simulink library "lib_converters"  (R2020b)
settings: Solver=VariableStepAuto  StartTime=0.0  StopTime=10.0  RelTol=1e-3
undefined symbols (not defined in the file): C_sc, DiscIntNeverNeededParam
libraries: powerlib x170, simulink x12, $bdroot x6, powerlib_meascontrol x3
(part 1 of 3)
settings Model: Creator=maloc  LastModifiedBy=maloc

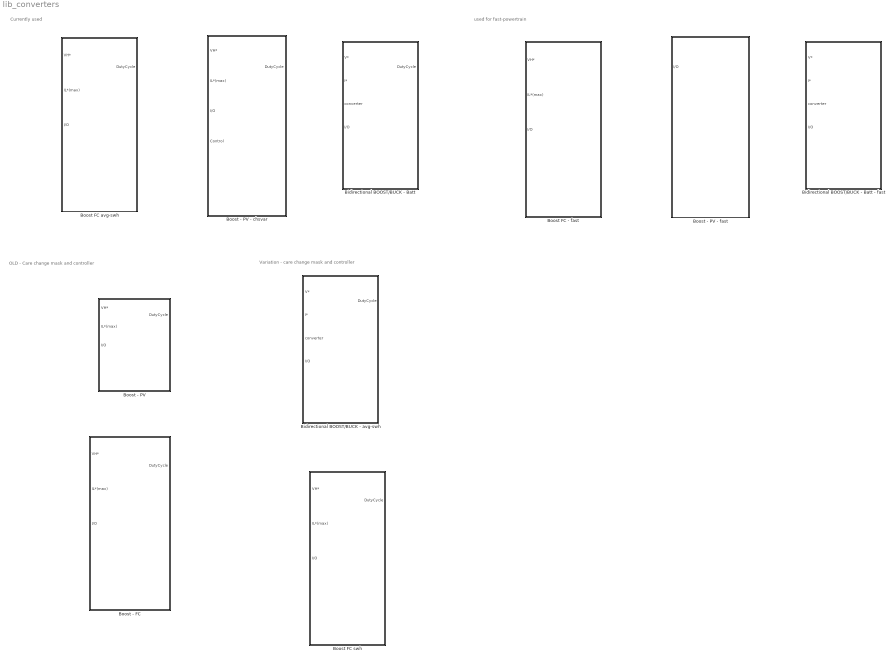
== system lib_converters ==
  note: Variation - care change mask and controller
  note: OLD - Care change mask and controller
  note: Currently used
  note: used for fast-powertrain
  Bidirectional BOOST/BUCK - Batt : Subsystem  mask(Average value DC/DC Bidirectional converter for Batt){n_buck=0.9, Tr_buck=1e-3, damp_buck=0, n_boost=0.9, Tr_boost=1e-3, damp_boost=0, max_curr=[45 -5], Co=1e-4, CL=1, Li=2e-3, Ts=1e-4}
      mask prompts: n_buck "Buck Efficiency [0,1]"; Tr_buck "Buck Regulator Response Time (s)"; damp_buck "Buck Damping ratio"; n_boost "Boost Efficiency [0,1]"; Tr_boost "Boost Regulator Response Time (s)"; damp_boost "Boost Damping ratio"; max_curr "Max currents [+ -] (A)"; Co "Capacitor (F)"; CL "DC Bus Capacitor (F)"; Li "Inductor (H)"; Ts "Sample Time (s)"
      mask help:
      | This block implements an average-value DC/DC Bidirectional boost/buck converter.
      | -> Boost
      | - V* is the voltage control variable. It controls the dc bus voltage (higher voltage part)
      | - I* is the current control variable. It controls the battery current (lower voltage part)
      |
      | <- Buck
      | - V* is the voltage control variable. It controls the battery voltage (lower voltage part)
      | - I* is the current control variable. It controls the current that comes from the dc bus (higher voltage part)
      |
      | - converter input controls the converter mode : 0 = Boost, 1 = Buck
      mask init:
      | L=Li; 
      | C=Co+CL;
      | 
      | 
      | 
      | %Buck :
      | %Current regulator
      | zetai_buck =damp_buck;
      | thau_si_buck =Tr_buck/10;
      | zetawni_buck=(-log(0.05*sqrt(1-zetai_buck^2)))/thau_si_buck;
      | Kpi_buck=2*L*zetawni_buck;
      | wni_buck=zetawni_buck/zetai_buck;
      | Kii_buck=L*wni_buck^2;
      |  
      | %Voltage regulator
      | zetav_buck=damp_buck;
      | thau_sv_buck=Tr_buck; %response time
      | zetawnv_buck=(-log(0.05*sqrt(1-zetav_buck^2)))/thau_sv_buck;
      | Kpv_buck=2*C*zetawnv_buck;
      | wnv_buck=zetawnv_buck/zetav_buck;
      | Kiv_buck=C*wnv_buck^2;
      | 
      | 
      | 
      | 
      | 
      | %Boost :
      | %Current regulator
      | zetai_boost=damp_boost;
      | thau_si_boost =Tr_boost/10; 
      | zetawni_boost =(-log(0.05*sqrt(1-zetai_boost ^2)))/thau_si_boost;
      | Kpi_boost=2*L*zetawni_boost;
      | wni_boost =zetawni_boost /zetai_boost;
      | Kii_boost=L*wni_boost ^2;
      |  
      | %Voltage regulator
      | zetav_boost =damp_boost;
      | thau_sv_boost =Tr_boost; %response time
      | zetawnv_boost =(-log(0.05*sqrt(1-zetav_boost ^2)))/thau_sv_boost;
      | Kpv_boost=2*C*zetawnv_boost;
      | wnv_boost =zetawnv_boost /zetav_boost;
      | Kiv_boost=C*wnv_boost ^2;
      mask Help:
      | 0 - Boost -->
      | <-- 1 - Buck
      mask DialogControl Container4 Prompt: Buck
      mask DialogControl Container5 Prompt: Boost
      mask DialogControl Container6 Prompt: All
  Bidirectional BOOST/BUCK - Batt - fast : Subsystem  AncestorBlock=lib_converters/Bidirectional BOOST//BUCK - Batt  mask(Average value DC/DC Bidirectional converter for Batt){n_buck=0.9, Tr_buck=1e-3, damp_buck=0, n_boost=0.9, Tr_boost=1e-3, damp_boost=0, max_curr=[45 -5], Co=1e-4, CL=1, Li=2e-3, Ts=1e-4}
      mask prompts: n_buck "Buck Efficiency [0,1]"; Tr_buck "Buck Regulator Response Time (s)"; damp_buck "Buck Damping ratio"; n_boost "Boost Efficiency [0,1]"; Tr_boost "Boost Regulator Response Time (s)"; damp_boost "Boost Damping ratio"; max_curr "Max currents [+ -] (A)"; Co "Capacitor (F)"; CL "DC Bus Capacitor (F)"; Li "Inductor (H)"; Ts "Sample Time (s)"
      mask help:
      | This block implements an average-value DC/DC Bidirectional boost/buck converter.
      | -> Boost
      | - V* is the voltage control variable. It controls the dc bus voltage (higher voltage part)
      | - I* is the current control variable. It controls the battery current (lower voltage part)
      |
      | <- Buck
      | - V* is the voltage control variable. It controls the battery voltage (lower voltage part)
      | - I* is the current control variable. It controls the current that comes from the dc bus (higher voltage part)
      |
      | - converter input controls the converter mode : 0 = Boost, 1 = Buck
      mask init: same as lib_converters/Bidirectional BOOST/BUCK - Batt
      mask Help:
      | 0 - Boost -->
      | <-- 1 - Buck
      mask DialogControl Container4 Prompt: Buck
      mask DialogControl Container5 Prompt: Boost
      mask DialogControl Container6 Prompt: All
  Bidirectional BOOST/BUCK - avg-swh : Subsystem  mask(Average value DC/DC Bidirectional converter for Batt){n_buck=0.9, Tr_buck=1e-3, n_boost=0.9, Tr_boost=1e-3, Co=1e-4, CL=1, Li=2e-3, Ts=1e-4}
      mask prompts: n_buck "Buck Efficiency [0,1]"; Tr_buck "Buck Regulator Response Time (s)"; n_boost "Boost Efficiency [0,1]"; Tr_boost "Boost Regulator Response Time (s)"; Co "Capacitor (F)"; CL "DC Bus Capacitor (F)"; Li "Inductor (H)"; Ts "Sample Time (s)"
      mask help:
      | This block implements an average-value DC/DC Bidirectional boost/buck converter.
      | -> Boost
      | - V* is the voltage control variable. It controls the dc bus voltage (higher voltage part)
      | - I* is the current control variable. It controls the battery current (lower voltage part)
      |
      | <- Buck
      | - V* is the voltage control variable. It controls the battery voltage (lower voltage part)
      | - I* is the current control variable. It controls the current that comes from the dc bus (higher voltage part)
      |
      | - converter input controls the converter mode : 0 = Boost, 1 = Buck
      mask init:
      | L=Li; 
      | C=Co+CL;
      | 
      | 
      | 
      | %Buck :
      | %Current regulator
      | zetai_buck =0.995;
      | % thau_si_buck =0.1/10; 
      | thau_si_buck =Tr_buck/10; 
      | zetawni_buck=(-log(0.05*sqrt(1-zetai_buck^2)))/thau_si_buck;
      | Kpi_buck=2*L*zetawni_buck;
      | wni_buck=zetawni_buck/zetai_buck;
      | Kii_buck=L*wni_buck^2;
      |  
      | %Voltage regulator
      | zetav_buck=0.995;
      | thau_sv_buck=Tr_buck; %response time
      | zetawnv_buck=(-log(0.05*sqrt(1-zetav_buck^2)))/thau_sv_buck;
      | Kpv_buck=2*C*zetawnv_buck;
      | wnv_buck=zetawnv_buck/zetav_buck;
      | Kiv_buck=C*wnv_buck^2;
      | 
      | 
      | 
      | 
      | 
      | %Boost :
      | %Current regulator
      | zetai_boost=0.707;
      | % thau_si_boost =0.1/10; 
      | thau_si_boost =Tr_boost/10; 
      | zetawni_boost =(-log(0.05*sqrt(1-zetai_boost ^2)))/thau_si_boost;
      | Kpi_boost=2*L*zetawni_boost;
      | wni_boost =zetawni_boost /zetai_boost;
      | Kii_boost=L*wni_boost ^2;
      |  
      | %Voltage regulator
      | zetav_boost =0.707;
      | thau_sv_boost =Tr_boost; %response time
      | zetawnv_boost =(-log(0.05*sqrt(1-zetav_boost ^2)))/thau_sv_boost;
      | Kpv_boost=2*C*zetawnv_boost;
      | wnv_boost =zetawnv_boost /zetav_boost;
      | Kiv_boost=C*wnv_boost ^2;
      mask Help:
      | 0 - Boost -->
      | <-- 1 - Buck
  Boost - FC : Subsystem  mask(Average value DC/DC boost converter for FC){n=0.9, Tr=1e-3, Co=100e-6, CL=1, Li=1e-3, Ts=1e-4}
      mask prompts: n "Efficiency [0,1]"; Tr "Response time (s) (Voltage Regulator)"; Co "Inside output capacitance (F)"; CL "Load Capacitance (F)"; Li "Input Inductor (H)"; Ts "Sample time (s)"
      mask help:
      | This block implements an average-value DC/DC boost converter.
      | - VH* input is the control variable of the output voltage of the converter.
      | - IL*(max) input is the control variable of the input max current of the converter.
      | - I/O input control the converter to enable it to work or not (interruptor control command).
      mask init:
      | L=Li; 
      | C=Co+CL;
      | 
      | %Current regulator
      | zetai=0.707;
      | % thau_si=0.1/10; 
      | thau_si=Tr/10; 
      | zetawni=(-log(0.05*sqrt(1-zetai^2)))/thau_si;
      | Kpi=2*L*zetawni;
      | wni=zetawni/zetai;
      | Kii=L*wni^2;
      | 
      | %Voltage regulator
      | zetav=0.707;
      | thau_sv=Tr; %response time
      | zetawnv=(-log(0.05*sqrt(1-zetav^2)))/thau_sv;
      | Kpv=2*C*zetawnv;
      | wnv=zetawnv/zetav;
      | Kiv=C*wnv^2;
  Boost - PV : Subsystem  mask(Average value DC/DC boost converter for PV panel){n=1, Tr=1e-3, Co=800e-5, CL=C_sc, Li=100e-5, Ts=1e-4, ControlType=MPPT}
      mask prompts: n "Efficiency [0,1]"; Tr "Response time (s) (Voltage Regulator)"; Co "Inside output capacitance (F)"; CL "Load Capacitance (F)"; Li "Input Inductor (H)"; Ts "Sample time (s)"; ControlType "Control of the converter"
      mask help:
      | This block implements an average-value DC/DC boost converter.
      | - VH* input is the control variable of the output voltage of the converter.
      | - IL*(max) input is the control variable of the input max current of the converter.
      | - I/O input control the converter to enable it to work or not (interruptor control command).
      |
      | Comment/Uncomment the wanted / unwanted control inside the block
      mask init:
      | L=Li; 
      | C=Co+CL;
      | 
      | %Current regulator
      | zetai=0.707;
      | thau_si=0.1/10; 
      | %zetawni=4.6/thau_si;
      | zetawni=(-log(0.05*sqrt(1-zetai^2)))/thau_si;
      | Kpi=2*L*zetawni;
      | wni=zetawni/zetai;
      | Kii=L*wni^2;
      | 
      | %Voltage regulator
      | zetav=0.707;
      | thau_sv=Tr; %response time
      | %zetawnv=4.6/thau_sv;
      | zetawnv=(-log(0.05*sqrt(1-zetav^2)))/thau_sv;
      | Kpv=2*C*zetawnv;
      | wnv=zetawnv/zetav;
      | Kiv=C*wnv^2;
      | 
      | 
      | %Choose between control type
      | SimulinkModel  = [gcb,'/Control'];
      | 
      | switch ControlType
      |     case 'MPPT'
      |         set_param(SimulinkModel,'OverrideUsingVariant','MPPT');
      |         
      |     case 'Cascade Control'
      |         set_param(SimulinkModel,'OverrideUsingVariant','Cascade-control');
      | end
      mask TypeOptions ControlType: MPPT | Cascade Control
      mask DialogControl Container3 Prompt: Control Type
  Boost - PV - chsvar : Subsystem  mask(Average value DC/DC boost converter for PV panel){n=1, Co=1e-4, CL=C_sc, Li=2e-3, damp=0.707, Tr=1e-3, Ts=1e-4}
      mask prompts: n "Efficiency [0,1]"; Co "Inside output capacitance (F)"; CL "Load Capacitance (F)"; Li "Input Inductor (H)"; damp "Damping ratio"; Tr "Response time (s) (Voltage Regulator)"; Ts "Sample time (s)"
      mask help:
      | This block implements an average-value DC/DC boost converter.
      | - VH* input is the control variable of the output voltage of the converter.
      | - IL*(max) input is the control variable of the input max current of the converter.
      | - I/O input control the converter to enable it to work or not (interruptor control command).
      | - Control input is the variable that manage the control strategy of the converter (MPPT, Cascade control, ...).
      mask init:
      | L=Li; 
      | C=Co+CL;
      | 
      | %Current regulator
      | zetai=damp;
      | thau_si=Tr/10;
      | zetawni=(-log(0.05*sqrt(1-zetai^2)))/thau_si;
      | Kpi=2*L*zetawni;
      | wni=zetawni/zetai;
      | Kii=L*wni^2;
      | 
      | %Voltage regulator
      | zetav=damp;
      | thau_sv=Tr; %response time
      | zetawnv=(-log(0.05*sqrt(1-zetav^2)))/thau_sv;
      | Kpv=2*C*zetawnv;
      | wnv=zetawnv/zetav;
      | Kiv=C*wnv^2;
      mask Help:
      | 1 - MPPT
      | 2 - Cascade control
  Boost - PV - fast : Subsystem  AncestorBlock=lib_converters/Boost - PV - chsvar  mask(Average value DC/DC boost converter for PV panel){n=1, Co=1e-4, CL=C_sc, Li=2e-3, damp=0.707, Tr=1e-3, Ts=1e-4}
      mask prompts: n "Efficiency [0,1]"; Co "Inside output capacitance (F)"; CL "Load Capacitance (F)"; Li "Input Inductor (H)"; damp "Damping ratio"; Tr "Response time (s) (Voltage Regulator)"; Ts "Sample time (s)"
      mask help:
      | This block implements an average-value DC/DC boost converter.
      | - VH* input is the control variable of the output voltage of the converter.
      | - IL*(max) input is the control variable of the input max current of the converter.
      | - I/O input control the converter to enable it to work or not (interruptor control command).
      | - Control input is the variable that manage the control strategy of the converter (MPPT, Cascade control, ...).
      mask init: same as lib_converters/Boost - PV - chsvar
      mask Help:
      | 1 - MPPT
      | 2 - Cascade control
  Boost FC - fast : Subsystem  AncestorBlock=lib_converters/Boost FC avg-swh  mask(Average value DC/DC boost converter for FC){conv_type=Average model, n=0.9, Co=1e-4, CL=1, Li=2e-3, damp=0.707, Tr=1e-3, Ts=1e-4}
      mask prompts: conv_type "Converter Type (dosen't work)"; n "Efficiency [0,1]"; Co "Inside output capacitance (F)"; CL "Load Capacitance (F)"; Li "Input Inductor (H)"; damp "Damping ratio"; Tr "Response time (s) (Voltage Regulator)"; Ts "Sample time (s)"
      mask help:
      | This block implements an average-value DC/DC boost converter.
      | - VH* input is the control variable of the output voltage of the converter.
      | - IL*(max) input is the control variable of the input max current of the converter.
      | - I/O input control the converter to enable it to work or not (interruptor control command).
      |
      | (To change the converter type you should go in the library, inside the block 'Boost FC avg-swh', right click on 'Converter Type' then 'Variant->Label' and choose the converter.
      mask init:
      | L=Li; 
      | C=Co+CL;
      | 
      | %Current regulator
      | zetai=damp;
      | thau_si=Tr/10; 
      | zetawni=(-log(0.05*sqrt(1-zetai^2)))/thau_si;
      | Kpi=2*L*zetawni;
      | wni=zetawni/zetai;
      | Kii=L*wni^2;
      | 
      | %Voltage regulator
      | zetav=damp;
      | thau_sv=Tr; %response time
      | zetawnv=(-log(0.05*sqrt(1-zetav^2)))/thau_sv;
      | Kpv=2*C*zetawnv;
      | wnv=zetawnv/zetav;
      | Kiv=C*wnv^2;
      | 
      | simmodel1 = [gcs,'/Boost FC avg-swh/Converter type'];
      | 
      | switch conv_type
      |     case 'Average model'
      |     set_param(simmodel1,'OverrideUsingVariant','Choice');
      |         case 'Switched model'
      |     set_param(simmodel1,'OverrideUsingVariant','Choice_1');
      | end
      mask TypeOptions conv_type: Average model | Switched model
  Boost FC avg-swh : Subsystem  mask(Average value DC/DC boost converter for FC){conv_type=Average model, n=0.9, Co=1e-4, CL=1, Li=2e-3, damp=0.707, Tr=1e-3, Ts=1e-4}
      mask prompts: conv_type "Converter Type (dosen't work)"; n "Efficiency [0,1]"; Co "Inside output capacitance (F)"; CL "Load Capacitance (F)"; Li "Input Inductor (H)"; damp "Damping ratio"; Tr "Response time (s) (Voltage Regulator)"; Ts "Sample time (s)"
      mask help:
      | This block implements an average-value DC/DC boost converter.
      | - VH* input is the control variable of the output voltage of the converter.
      | - IL*(max) input is the control variable of the input max current of the converter.
      | - I/O input control the converter to enable it to work or not (interruptor control command).
      |
      | (To change the converter type you should go in the library, inside the block 'Boost FC avg-swh', right click on 'Converter Type' then 'Variant->Label' and choose the converter.
      mask init: same as lib_converters/Boost FC - fast
      mask TypeOptions conv_type: Average model | Switched model
  Boost FC swh : Subsystem  mask(Average value DC/DC boost converter for FC){conv_type=Switched model, n=0.9, Tr=1e-3, Co=1e-4, CL=1, Li=2e-3, Ts=1e-4}
      mask prompts: conv_type "Converter Type (dosen't work)"; n "Efficiency [0,1]"; Tr "Response time (s) (Voltage Regulator)"; Co "Inside output capacitance (F)"; CL "Load Capacitance (F)"; Li "Input Inductor (H)"; Ts "Sample time (s)"
      mask help:
      | This block implements an average-value DC/DC boost converter.
      | - VH* input is the control variable of the output voltage of the converter.
      | - IL*(max) input is the control variable of the input max current of the converter.
      | - I/O input control the converter to enable it to work or not (interruptor control command).
      |
      | (To change the converter type you should go in the library, inside the block 'Boost FC avg-swh', right click on 'Converter Type' then 'Variant->Label' and choose the converter.
      mask init:
      | L=Li; 
      | C=Co+CL;
      | 
      | %Current regulator
      | zetai=0.707;
      | % thau_si=0.1/10; 
      | thau_si=Tr/10; 
      | zetawni=(-log(0.05*sqrt(1-zetai^2)))/thau_si;
      | Kpi=2*L*zetawni;
      | wni=zetawni/zetai;
      | Kii=L*wni^2;
      | 
      | %Voltage regulator
      | zetav=0.707;
      | thau_sv=Tr; %response time
      | zetawnv=(-log(0.05*sqrt(1-zetav^2)))/thau_sv;
      | Kpv=2*C*zetawnv;
      | wnv=zetawnv/zetav;
      | Kiv=C*wnv^2;
      | 
      | simmodel1 = [gcs,'/Boost FC avg-swh/Converter type'];
      | 
      | switch conv_type
      |     case 'Average model'
      |     set_param(simmodel1,'OverrideUsingVariant','Choice');
      |         case 'Switched model'
      |     set_param(simmodel1,'OverrideUsingVariant','Choice_1');
      | end
      mask TypeOptions conv_type: Average model | Switched model

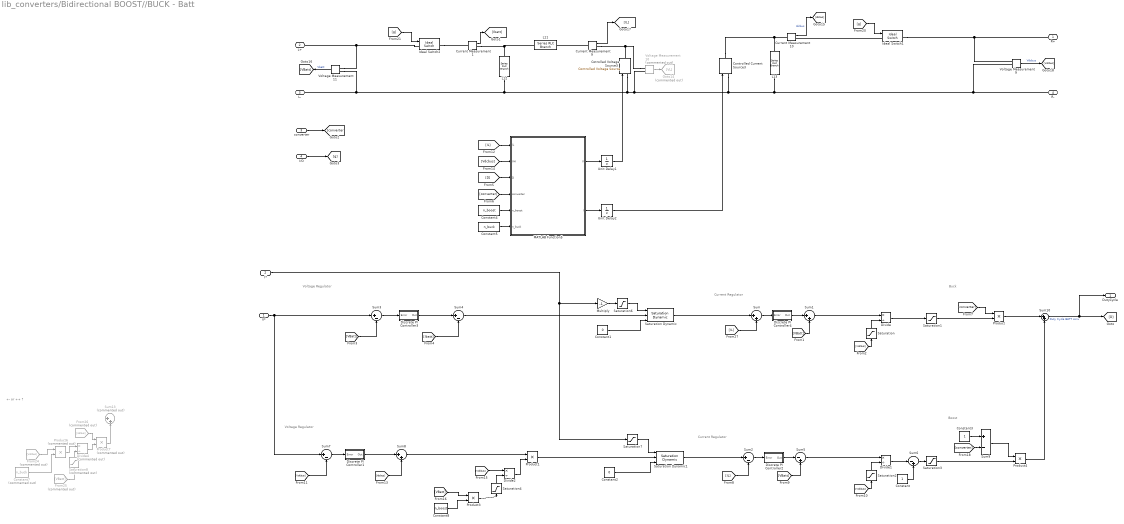
== system lib_converters/Bidirectional BOOST//BUCK - Batt ==
  note: Boost
  note: Buck
  note: Voltage Regulator
  note: Current Regulator
  note: Voltage Regulator
  note: Current Regulator
  note: +- or ++ ?
  V* : Inport
  I* : Inport  Port=2
  converter : Inport  Port=3
  I/O : Inport  Port=4
  Constant : Constant
  Constant1 : Constant  Value=0
  Constant2 : Constant  Value=0
  Constant3 : Constant
  Constant4 : Constant  Value=n_boost
  Constant5 : Constant  Value=n_buck
  Constant7 : Constant  Commented=on  Value=n_buck
  Constant8 : Constant  Value=n_boost
  Controlled Current Source3 : powerlib/Electrical Sources/Controlled Current Source  Initialize=on  Source_Type=DC  Amplitude=0  Phase=0  Frequency=0  Measurements=None
  Cotrolled Voltage Source3 : powerlib/Electrical Sources/Controlled Voltage Source  Initialize=on  Source_Type=DC  Amplitude=0  Phase=0  Frequency=0  Measurements=None
  Current Measurement1 : powerlib/Measurements/Current Measurement  PhasorSimulation=off  OutputType=Complex  PSBequivalent=0
  Current Measurement10 : powerlib/Measurements/Current Measurement  PhasorSimulation=off  OutputType=Complex  PSBequivalent=0
  Current Measurement9 : powerlib/Measurements/Current Measurement  PhasorSimulation=off  OutputType=Complex  PSBequivalent=0
  Discrete PI Controller1 : Subsystem  DialogController=POWERSYS.PowerSysDialog  mask(Discrete PI Controller){Kp=Kpv_boost, Ki=Kiv_boost, Par_Limits=[0.5 -0.5], Init=0, Ts=Ts}
      mask prompts: Kp "Proportional gain (Kp):"; Ki "Integral gain (Ki):"; Par_Limits "Output limits: [ Upper   Lower ]"; Init "Output initial value:"; Ts "Sample time:"
      mask help: This block implements a discrete PI controller.
      mask init:
      | UpperLimit=Par_Limits(1);
      | LowerLimit=Par_Limits(2);
      | power_initmask();
      mask Help: This block is part of a subset of blocks in the Extras library that does not have documentation associated with it, other than the block mask description.
      mask Display: disp('PI');
  Discrete PI Controller2 : Subsystem  DialogController=POWERSYS.PowerSysDialog  mask(Discrete PI Controller){Kp=Kpi_boost, Ki=Kii_boost, Par_Limits=[50 -50], Init=0, Ts=Ts}
      mask prompts: Kp "Proportional gain (Kp):"; Ki "Integral gain (Ki):"; Par_Limits "Output limits: [ Upper   Lower ]"; Init "Output initial value:"; Ts "Sample time:"
      mask help: This block implements a discrete PI controller.
      mask init:
      | UpperLimit=Par_Limits(1);
      | LowerLimit=Par_Limits(2);
      | power_initmask();
      mask Help: This block is part of a subset of blocks in the Extras library that does not have documentation associated with it, other than the block mask description.
      mask Display: disp('PI');
  Discrete PI Controller3 : Subsystem  DialogController=POWERSYS.PowerSysDialog  mask(Discrete PI Controller){Kp=Kpv_buck, Ki=Kiv_buck, Par_Limits=[1 -1], Init=0, Ts=Ts}
      mask prompts: Kp "Proportional gain (Kp):"; Ki "Integral gain (Ki):"; Par_Limits "Output limits: [ Upper   Lower ]"; Init "Output initial value:"; Ts "Sample time:"
      mask help: This block implements a discrete PI controller.
      mask init:
      | UpperLimit=Par_Limits(1);
      | LowerLimit=Par_Limits(2);
      | power_initmask();
      mask Help: This block is part of a subset of blocks in the Extras library that does not have documentation associated with it, other than the block mask description.
      mask Display: disp('PI');
  Discrete PI Controller4 : Subsystem  DialogController=POWERSYS.PowerSysDialog  mask(Discrete PI Controller){Kp=Kpi_buck, Ki=Kii_buck, Par_Limits=[1 -1], Init=0, Ts=Ts}
      mask prompts: Kp "Proportional gain (Kp):"; Ki "Integral gain (Ki):"; Par_Limits "Output limits: [ Upper   Lower ]"; Init "Output initial value:"; Ts "Sample time:"
      mask help: This block implements a discrete PI controller.
      mask init:
      | UpperLimit=Par_Limits(1);
      | LowerLimit=Par_Limits(2);
      | power_initmask();
      mask Help: This block is part of a subset of blocks in the Extras library that does not have documentation associated with it, other than the block mask description.
      mask Display: disp('PI');
  Divide : Product  Inputs=*/  SampleTime=Ts
  Divide1 : Product  Inputs=*/  SampleTime=Ts
  Divide2 : Product  Inputs=*/  SampleTime=Ts
  Divide4 : Product  Commented=on  Inputs=*/  SampleTime=Ts
  From24 : From  Commented=on  GotoTag=Vdcbus
  From25 : From  Commented=on  GotoTag=VBatt
  From26 : From  Commented=on  GotoTag=Idcbus
  Goto14 : Goto  Commented=on  GotoTag=VL
  Ideal Switch1 : powerlib/Power Electronics/Ideal Switch  Ron=0.001  Lon=0  IC=0  Rs=1e5  Cs=inf  Measurements=off
  Ideal Switch2 : powerlib/Power Electronics/Ideal Switch  Ron=0.001  Lon=0  IC=0  Rs=1e5  Cs=inf  Measurements=off
  L11 : powerlib/Elements/Series RLC Branch  LConnTagsString=__new0  RConnTagsString=__new0  BranchType=L  Resistance=0.3  Inductance=L  SetiL0=off  InitialCurrent=100  Capacitance=100e-6  Setx0=off  InitialVoltage=0  Measurements=None
  L12 : powerlib/Elements/Series RLC Branch  LConnTagsString=__new0  RConnTagsString=__new0  BranchType=RC  Resistance=0.01  Inductance=100e-6  SetiL0=off  InitialCurrent=100  Capacitance=Co  Setx0=off  InitialVoltage=0  Measurements=None
  L13 : powerlib/Elements/Series RLC Branch  LConnTagsString=__new0  RConnTagsString=__new0  BranchType=RC  Resistance=0.01  Inductance=100e-6  SetiL0=off  InitialCurrent=100  Capacitance=Co  Setx0=off  InitialVoltage=0  Measurements=None
  MATLAB Function5 : MATLAB Function  TreatAsAtomicUnit=on
  Multiply : Gain  Gain=-1
  Product : Product
  Product1 : Product  RndMeth=Zero
  Product3 : Product  RndMeth=Zero
  Product4 : Product
  Product6 : Product  Commented=on  RndMeth=Zero
  Product7 : Product  Commented=on  RndMeth=Zero
  Saturation : Saturate  UpperLimit=inf  LowerLimit=0.01  SampleTime=Ts
  Saturation Dynamic : simulink/Discontinuities/Saturation Dynamic  OutMin=[]  OutMax=[]  OutDataTypeStr=Inherit: Same as second input  OutDataType=fixdt(1, 16)  OutScaling=2^-10  DoSatur=off
  Saturation Dynamic1 : simulink/Discontinuities/Saturation Dynamic  OutMin=[]  OutMax=[]  OutDataTypeStr=Inherit: Same as second input  OutDataType=fixdt(1, 16)  OutScaling=2^-10  DoSatur=off
  Saturation1 : Saturate  UpperLimit=1  LowerLimit=0  SampleTime=Ts
  Saturation2 : Saturate  UpperLimit=inf  LowerLimit=0.01  SampleTime=Ts
  Saturation3 : Saturate  UpperLimit=1  LowerLimit=0  SampleTime=Ts
  Saturation4 : Saturate  UpperLimit=inf  LowerLimit=0.01  SampleTime=Ts
  Saturation6 : Saturate  UpperLimit=-max_curr(2)  LowerLimit=0
  Saturation7 : Saturate  UpperLimit=max_curr(1)  LowerLimit=0
  Saturation8 : Saturate  Commented=on  UpperLimit=inf  LowerLimit=0.01  SampleTime=Ts
  Sum{,1,8,10} (4 alike) : Sum  Inputs=|++
  Sum13 : Sum  Commented=on  Inputs=|++
  Sum{2..4,7} (4 alike) : Sum  Inputs=|+-
  Sum5 : Sum  Inputs=|-+
  Sum6 : Sum  Inputs=|-+
  Sum9 : Sum  Inputs=+-
  Unit Delay1 : UnitDelay  SampleTime=Ts  HasFrameUpgradeWarning=on
  Unit Delay2 : UnitDelay  SampleTime=Ts  HasFrameUpgradeWarning=on
  Voltage Measurement10 : powerlib/Measurements/Voltage Measurement  Commented=on  PhasorSimulation=off  OutputType=Complex  PSBequivalent=0
  Voltage Measurement11 : powerlib/Measurements/Voltage Measurement  PhasorSimulation=off  OutputType=Complex  PSBequivalent=0
  Voltage Measurement9 : powerlib/Measurements/Voltage Measurement  PhasorSimulation=off  OutputType=Complex  PSBequivalent=0
  R+ : PMIOPort  Side=Right
  L+ : PMIOPort  Port=2  Side=Left
  L- : PMIOPort  Port=3  Side=Left
  R- : PMIOPort  Port=4  Side=Right
  DutyCycle : Outport
  wires:
  I*/1 -> Multiply/1, Saturation7/1
  Saturation7/1 -> Saturation Dynamic1/1
  Saturation6/1 -> Saturation Dynamic/1
  Multiply/1 -> Saturation6/1
  Sum10/1 -> [D], DutyCycle/1  "Duty Cycle BATT conv"
  Product4/1 -> Sum10/2
  Product/1 -> Sum10/1
  Sum9/1 -> Product4/1
  [converter] -> Sum9/2
  Constant3/1 -> Sum9/1
  Saturation3/1 -> Product4/2
  Saturation4/1 -> Divide2/2
  Saturation2/1 -> Divide1/2
  Divide1/1 -> Sum6/1
  Discrete PI Controller2/1(Out) -> Sum5/1
  Constant8/1 -> Product3/2
  [Idcbus] -> Sum8/2
  Discrete PI Controller1/1(Out) -> Sum8/1
  Sum6/1 -> Saturation3/1
  Product1/1 -> Saturation Dynamic1/2
  Sum8/1 -> Product1/1
  V*/1 -> Sum3/1, Sum7/1
  [VBatt] -> Product3/1
  Product3/1 -> Saturation4/1
  Sum7/1 -> Discrete PI Controller1/1(Error)
  Divide2/1 -> Product1/2
  [Vdcbus] -> Sum7/2
  Constant2/1 -> Saturation Dynamic1/3
  Saturation Dynamic1/1 -> Sum2/1
  [Vdcbus] -> Divide2/1
  Sum5/1 -> Divide1/1
  [VBatt] -> Sum5/2
  Constant/1 -> Sum6/2
  Sum2/1 -> Discrete PI Controller2/1(Error)
  [IL] -> Sum2/2
  [Vdcbus] -> Saturation2/1
  [converter] -> Product/1
  [converter] -> MATLAB Function5/4(converter)
  converter/1 -> [converter]
  Saturation1/1 -> Product/2
  Current Measurement1/1 -> [Ibatt]
  Sum1/1 -> Divide/1
  [Vdcbus] -> Saturation/1
  Divide/1 -> Saturation1/1
  [VBatt] -> Sum1/2
  Sum4/1 -> Saturation Dynamic/2
  Constant1/1 -> Saturation Dynamic/3
  Discrete PI Controller4/1(Out) -> Sum1/1
  Saturation/1 -> Divide/2
  [VBatt] -> Sum3/2
  Sum/1 -> Discrete PI Controller4/1(Error)
  Saturation Dynamic/1 -> Sum/1
  Sum3/1 -> Discrete PI Controller3/1(Error)
  Current Measurement9/1 -> [IL]
  Unit Delay1/1 -> Cotrolled Voltage Source3/1
  Voltage Measurement10/1 -> Goto14/1
  Voltage Measurement9/1 -> [Vdcbus]  "Vdcbus"
  Unit Delay2/1 -> Controlled Current Source3/1
  Current Measurement10/1 -> [Idcbus]  "Idcbus"
  [D] -> MATLAB Function5/3(D)
  [IL] -> MATLAB Function5/1(iL)
  Voltage Measurement11/1 -> [VBatt]  "Vbatt"
  [Vdcbus] -> MATLAB Function5/2(VH)
  [g] -> Ideal Switch1/1
  [g] -> Ideal Switch2/1
  I/O/1 -> [g]
  MATLAB Function5/1(V) -> Unit Delay1/1
  MATLAB Function5/2(I) -> Unit Delay2/1
  Constant4/1 -> MATLAB Function5/5(n_boost)
  Constant5/1 -> MATLAB Function5/6(n_buck)
  Discrete PI Controller3/1(Out) -> Sum4/1
  Product6/1 -> Divide4/1
  From24/1 -> Product6/1
  From26/1 -> Product7/1
  Divide4/1 -> Product7/2
  Product7/1 -> Sum13/2
  From25/1 -> Saturation8/1
  Constant7/1 -> Product6/2
  Saturation8/1 -> Divide4/2
  [Ibatt] -> Sum4/2
  [IL] -> Sum/2
  connections:
  Current Measurement1/RConn1 -- L11/RConn1 -- L12/LConn1
  Controlled Current Source3/RConn1 -- L13/LConn1 -- Current Measurement10/LConn1
  R+/RConn1 -- Voltage Measurement9/LConn1 -- Ideal Switch1/RConn1
  Voltage Measurement10/LConn1 -- Current Measurement9/RConn1 -- Cotrolled Voltage Source3/RConn1
  Current Measurement9/LConn1 -- L11/LConn1
  Voltage Measurement11/LConn2 -- Voltage Measurement9/LConn2 -- R-/RConn1 -- L13/RConn1 -- Controlled Current Source3/LConn1 -- Voltage Measurement10/LConn2 -- Cotrolled Voltage Source3/LConn1 -- L12/RConn1 -- L-/RConn1
  Ideal Switch1/LConn1 -- Current Measurement10/RConn1
  Voltage Measurement11/LConn1 -- L+/RConn1 -- Ideal Switch2/LConn1
  Ideal Switch2/RConn1 -- Current Measurement1/LConn1

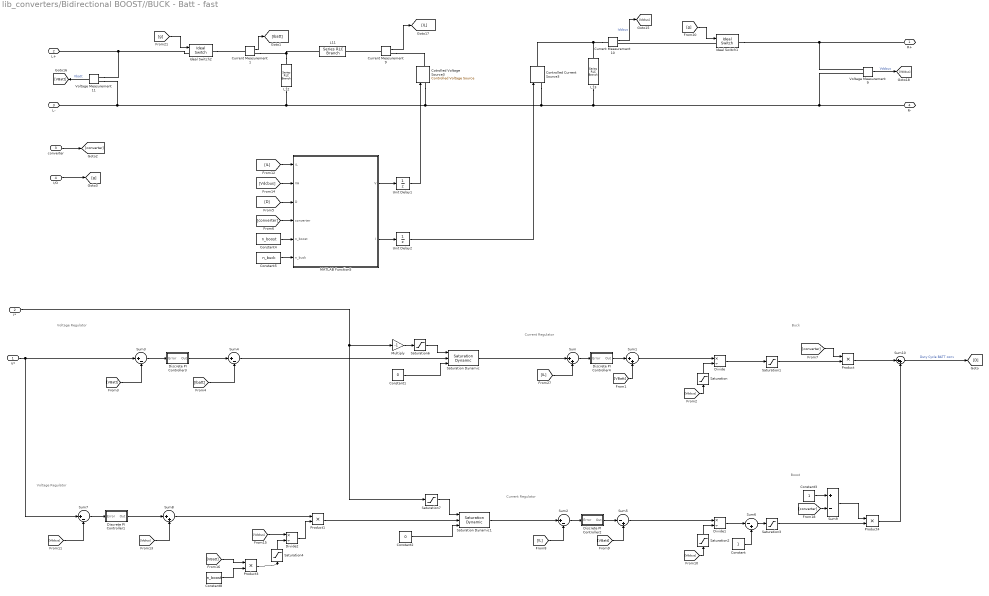
== system lib_converters/Bidirectional BOOST//BUCK - Batt - fast ==
  note: Current Regulator
  note: Voltage Regulator
  note: Current Regulator
  note: Voltage Regulator
  note: Buck
  note: Boost
  V* : Inport
  I* : Inport  Port=2
  converter : Inport  Port=3
  I/O : Inport  Port=4
  Constant : Constant
  Constant1 : Constant  Value=0
  Constant2 : Constant  Value=0
  Constant3 : Constant
  Constant4 : Constant  Value=n_boost
  Constant5 : Constant  Value=n_buck
  Constant8 : Constant  Value=n_boost
  Controlled Current Source3 : powerlib/Electrical Sources/Controlled Current Source  Initialize=on  Source_Type=DC  Amplitude=0  Phase=0  Frequency=0  Measurements=None
  Cotrolled Voltage Source3 : powerlib/Electrical Sources/Controlled Voltage Source  Initialize=on  Source_Type=DC  Amplitude=0  Phase=0  Frequency=0  Measurements=None
  Current Measurement1 : powerlib/Measurements/Current Measurement  PhasorSimulation=off  OutputType=Complex  PSBequivalent=0
  Current Measurement10 : powerlib/Measurements/Current Measurement  PhasorSimulation=off  OutputType=Complex  PSBequivalent=0
  Current Measurement9 : powerlib/Measurements/Current Measurement  PhasorSimulation=off  OutputType=Complex  PSBequivalent=0
  Discrete PI Controller1 : Subsystem  DialogController=POWERSYS.PowerSysDialog  mask(Discrete PI Controller){Kp=Kpv_boost, Ki=Kiv_boost, Par_Limits=[0.5 -0.5], Init=0, Ts=Ts}
      mask prompts: Kp "Proportional gain (Kp):"; Ki "Integral gain (Ki):"; Par_Limits "Output limits: [ Upper   Lower ]"; Init "Output initial value:"; Ts "Sample time:"
      mask help: This block implements a discrete PI controller.
      mask init:
      | UpperLimit=Par_Limits(1);
      | LowerLimit=Par_Limits(2);
      | power_initmask();
      mask Help: This block is part of a subset of blocks in the Extras library that does not have documentation associated with it, other than the block mask description.
      mask Display: disp('PI');
  Discrete PI Controller2 : Subsystem  DialogController=POWERSYS.PowerSysDialog  mask(Discrete PI Controller){Kp=Kpi_boost, Ki=Kii_boost, Par_Limits=[50 -50], Init=0, Ts=Ts}
      mask prompts: Kp "Proportional gain (Kp):"; Ki "Integral gain (Ki):"; Par_Limits "Output limits: [ Upper   Lower ]"; Init "Output initial value:"; Ts "Sample time:"
      mask help: This block implements a discrete PI controller.
      mask init:
      | UpperLimit=Par_Limits(1);
      | LowerLimit=Par_Limits(2);
      | power_initmask();
      mask Help: This block is part of a subset of blocks in the Extras library that does not have documentation associated with it, other than the block mask description.
      mask Display: disp('PI');
  Discrete PI Controller3 : Subsystem  DialogController=POWERSYS.PowerSysDialog  mask(Discrete PI Controller){Kp=Kpv_buck, Ki=Kiv_buck, Par_Limits=[1 -1], Init=0, Ts=Ts}
      mask prompts: Kp "Proportional gain (Kp):"; Ki "Integral gain (Ki):"; Par_Limits "Output limits: [ Upper   Lower ]"; Init "Output initial value:"; Ts "Sample time:"
      mask help: This block implements a discrete PI controller.
      mask init:
      | UpperLimit=Par_Limits(1);
      | LowerLimit=Par_Limits(2);
      | power_initmask();
      mask Help: This block is part of a subset of blocks in the Extras library that does not have documentation associated with it, other than the block mask description.
      mask Display: disp('PI');
  Discrete PI Controller4 : Subsystem  DialogController=POWERSYS.PowerSysDialog  mask(Discrete PI Controller){Kp=Kpi_buck, Ki=Kii_buck, Par_Limits=[1 -1], Init=0, Ts=Ts}
      mask prompts: Kp "Proportional gain (Kp):"; Ki "Integral gain (Ki):"; Par_Limits "Output limits: [ Upper   Lower ]"; Init "Output initial value:"; Ts "Sample time:"
      mask help: This block implements a discrete PI controller.
      mask init:
      | UpperLimit=Par_Limits(1);
      | LowerLimit=Par_Limits(2);
      | power_initmask();
      mask Help: This block is part of a subset of blocks in the Extras library that does not have documentation associated with it, other than the block mask description.
      mask Display: disp('PI');
  Divide : Product  Inputs=*/  SampleTime=Ts
  Divide1 : Product  Inputs=*/  SampleTime=Ts
  Divide2 : Product  Inputs=*/  SampleTime=Ts
  Ideal Switch1 : powerlib/Power Electronics/Ideal Switch  Ron=0.001  Lon=0  IC=0  Rs=1e5  Cs=inf  Measurements=off
  Ideal Switch2 : powerlib/Power Electronics/Ideal Switch  Ron=0.001  Lon=0  IC=0  Rs=1e5  Cs=inf  Measurements=off
  L11 : powerlib/Elements/Series RLC Branch  LConnTagsString=__new0  RConnTagsString=__new0  BranchType=L  Resistance=0.3  Inductance=L  SetiL0=off  InitialCurrent=100  Capacitance=100e-6  Setx0=off  InitialVoltage=0  Measurements=None
  L12 : powerlib/Elements/Series RLC Branch  LConnTagsString=__new0  RConnTagsString=__new0  BranchType=RC  Resistance=0.01  Inductance=100e-6  SetiL0=off  InitialCurrent=100  Capacitance=Co  Setx0=off  InitialVoltage=0  Measurements=None
  L13 : powerlib/Elements/Series RLC Branch  LConnTagsString=__new0  RConnTagsString=__new0  BranchType=RC  Resistance=0.01  Inductance=100e-6  SetiL0=off  InitialCurrent=100  Capacitance=Co  Setx0=off  InitialVoltage=0  Measurements=None
  MATLAB Function5 : MATLAB Function  TreatAsAtomicUnit=on
  Multiply : Gain  Gain=-1
  Product : Product
  Product1 : Product  RndMeth=Zero
  Product3 : Product  RndMeth=Zero
  Product4 : Product
  Saturation : Saturate  UpperLimit=inf  LowerLimit=0.01  SampleTime=Ts
  Saturation Dynamic : simulink/Discontinuities/Saturation Dynamic  OutMin=[]  OutMax=[]  OutDataTypeStr=Inherit: Same as second input  OutDataType=fixdt(1, 16)  OutScaling=2^-10  DoSatur=off
  Saturation Dynamic1 : simulink/Discontinuities/Saturation Dynamic  OutMin=[]  OutMax=[]  OutDataTypeStr=Inherit: Same as second input  OutDataType=fixdt(1, 16)  OutScaling=2^-10  DoSatur=off
  Saturation1 : Saturate  UpperLimit=1  LowerLimit=0  SampleTime=Ts
  Saturation2 : Saturate  UpperLimit=inf  LowerLimit=0.01  SampleTime=Ts
  Saturation3 : Saturate  UpperLimit=1  LowerLimit=0  SampleTime=Ts
  Saturation4 : Saturate  UpperLimit=inf  LowerLimit=0.01  SampleTime=Ts
  Saturation6 : Saturate  UpperLimit=-max_curr(2)  LowerLimit=0
  Saturation7 : Saturate  UpperLimit=max_curr(1)  LowerLimit=0
  Sum{,1,8,10} (4 alike) : Sum  Inputs=|++
  Sum{2..4,7} (4 alike) : Sum  Inputs=|+-
  Sum5 : Sum  Inputs=|-+
  Sum6 : Sum  Inputs=|-+
  Sum9 : Sum  Inputs=+-
  Unit Delay1 : UnitDelay  SampleTime=Ts  HasFrameUpgradeWarning=on
  Unit Delay2 : UnitDelay  SampleTime=Ts  HasFrameUpgradeWarning=on
  Voltage Measurement11 : powerlib/Measurements/Voltage Measurement  PhasorSimulation=off  OutputType=Complex  PSBequivalent=0
  Voltage Measurement9 : powerlib/Measurements/Voltage Measurement  PhasorSimulation=off  OutputType=Complex  PSBequivalent=0
  R+ : PMIOPort  Side=Right
  L+ : PMIOPort  Port=2  Side=Left
  L- : PMIOPort  Port=3  Side=Left
  R- : PMIOPort  Port=4  Side=Right
  wires:
  [IL] -> Sum/2
  [Ibatt] -> Sum4/2
  Discrete PI Controller3/1(Out) -> Sum4/1
  Constant5/1 -> MATLAB Function5/6(n_buck)
  Constant4/1 -> MATLAB Function5/5(n_boost)
  MATLAB Function5/2(I) -> Unit Delay2/1
  MATLAB Function5/1(V) -> Unit Delay1/1
  I/O/1 -> [g]
  [g] -> Ideal Switch2/1
  [g] -> Ideal Switch1/1
  [Vdcbus] -> MATLAB Function5/2(VH)
  Voltage Measurement11/1 -> [VBatt]  "Vbatt"
  [IL] -> MATLAB Function5/1(iL)
  [D] -> MATLAB Function5/3(D)
  Current Measurement10/1 -> [Idcbus]  "Idcbus"
  Unit Delay2/1 -> Controlled Current Source3/1
  Voltage Measurement9/1 -> [Vdcbus]  "Vdcbus"
  Unit Delay1/1 -> Cotrolled Voltage Source3/1
  Current Measurement9/1 -> [IL]
  Sum3/1 -> Discrete PI Controller3/1(Error)
  Saturation Dynamic/1 -> Sum/1
  Sum/1 -> Discrete PI Controller4/1(Error)
  [VBatt] -> Sum3/2
  Saturation/1 -> Divide/2
  Discrete PI Controller4/1(Out) -> Sum1/1
  Constant1/1 -> Saturation Dynamic/3
  Sum4/1 -> Saturation Dynamic/2
  [VBatt] -> Sum1/2
  Divide/1 -> Saturation1/1
  [Vdcbus] -> Saturation/1
  Sum1/1 -> Divide/1
  Current Measurement1/1 -> [Ibatt]
  Saturation1/1 -> Product/2
  converter/1 -> [converter]
  [converter] -> MATLAB Function5/4(converter)
  [converter] -> Product/1
  [Vdcbus] -> Saturation2/1
  [IL] -> Sum2/2
  Sum2/1 -> Discrete PI Controller2/1(Error)
  Constant/1 -> Sum6/2
  [VBatt] -> Sum5/2
  Sum5/1 -> Divide1/1
  [Vdcbus] -> Divide2/1
  Saturation Dynamic1/1 -> Sum2/1
  Constant2/1 -> Saturation Dynamic1/3
  [Vdcbus] -> Sum7/2
  Divide2/1 -> Product1/2
  Sum7/1 -> Discrete PI Controller1/1(Error)
  Product3/1 -> Saturation4/1
  [VBatt] -> Product3/1
  V*/1 -> Sum7/1, Sum3/1
  Sum8/1 -> Product1/1
  Product1/1 -> Saturation Dynamic1/2
  Sum6/1 -> Saturation3/1
  Discrete PI Controller1/1(Out) -> Sum8/1
  [Idcbus] -> Sum8/2
  Constant8/1 -> Product3/2
  Discrete PI Controller2/1(Out) -> Sum5/1
  Divide1/1 -> Sum6/1
  Saturation2/1 -> Divide1/2
  Saturation4/1 -> Divide2/2
  Saturation3/1 -> Product4/2
  Constant3/1 -> Sum9/1
  [converter] -> Sum9/2
  Sum9/1 -> Product4/1
  Product/1 -> Sum10/1
  Product4/1 -> Sum10/2
  Sum10/1 -> [D]  "Duty Cycle BATT conv"
  Multiply/1 -> Saturation6/1
  Saturation6/1 -> Saturation Dynamic/1
  Saturation7/1 -> Saturation Dynamic1/1
  I*/1 -> Saturation7/1, Multiply/1
  connections:
  Ideal Switch2/RConn1 -- Current Measurement1/LConn1
  Ideal Switch2/LConn1 -- L+/RConn1 -- Voltage Measurement11/LConn1
  Ideal Switch1/LConn1 -- Current Measurement10/RConn1
  L-/RConn1 -- L12/RConn1 -- Controlled Current Source3/LConn1 -- L13/RConn1 -- R-/RConn1 -- Voltage Measurement9/LConn2 -- Cotrolled Voltage Source3/LConn1 -- Voltage Measurement11/LConn2
  Current Measurement9/LConn1 -- L11/LConn1
  Current Measurement9/RConn1 -- Cotrolled Voltage Source3/RConn1
  Ideal Switch1/RConn1 -- Voltage Measurement9/LConn1 -- R+/RConn1
  Current Measurement10/LConn1 -- L13/LConn1 -- Controlled Current Source3/RConn1
  L12/LConn1 -- L11/RConn1 -- Current Measurement1/RConn1

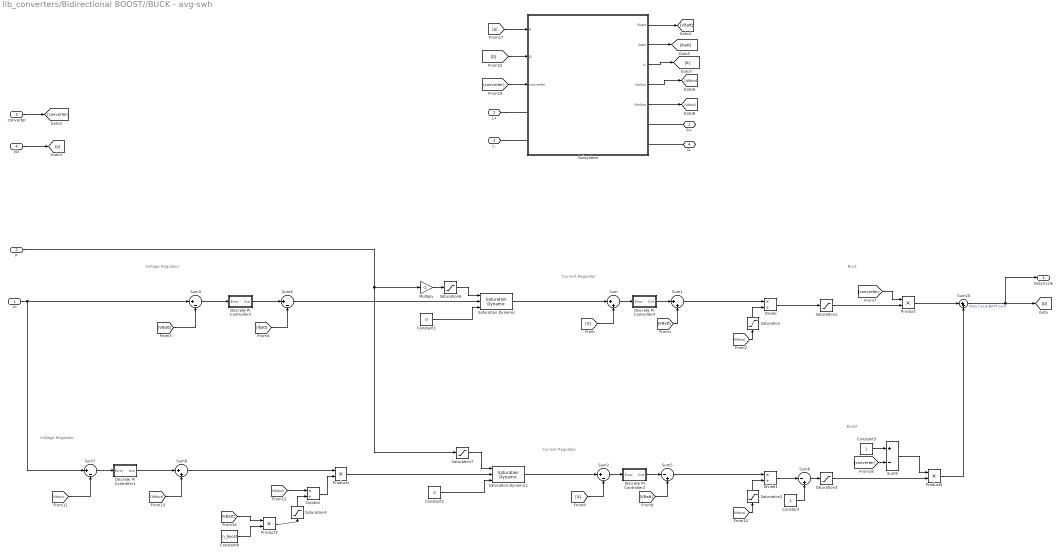
== system lib_converters/Bidirectional BOOST//BUCK - avg-swh ==
  note: Current Regulator
  note: Voltage Regulator
  note: Current Regulator
  note: Voltage Regulator
  note: Buck
  note: Boost
  V* : Inport
  I* : Inport  Port=2
  converter : Inport  Port=3
  I/O : Inport  Port=4
  Constant : Constant
  Constant1 : Constant  Value=0
  Constant2 : Constant  Value=0
  Constant3 : Constant
  Constant8 : Constant  Value=n_boost
  Discrete PI Controller1 : Subsystem  DialogController=POWERSYS.PowerSysDialog  mask(Discrete PI Controller){Kp=Kpv_boost, Ki=Kiv_boost, Par_Limits=[0.5 -0.5], Init=0, Ts=Tr_boost}
      mask prompts: Kp "Proportional gain (Kp):"; Ki "Integral gain (Ki):"; Par_Limits "Output limits: [ Upper   Lower ]"; Init "Output initial value:"; Ts "Sample time:"
      mask help: This block implements a discrete PI controller.
      mask init:
      | UpperLimit=Par_Limits(1);
      | LowerLimit=Par_Limits(2);
      | power_initmask();
      mask Help: This block is part of a subset of blocks in the Extras library that does not have documentation associated with it, other than the block mask description.
      mask Display: disp('PI');
  Discrete PI Controller2 : Subsystem  DialogController=POWERSYS.PowerSysDialog  mask(Discrete PI Controller){Kp=Kpi_boost, Ki=Kii_boost, Par_Limits=[50 -50], Init=0, Ts=Ts}
      mask prompts: Kp "Proportional gain (Kp):"; Ki "Integral gain (Ki):"; Par_Limits "Output limits: [ Upper   Lower ]"; Init "Output initial value:"; Ts "Sample time:"
      mask help: This block implements a discrete PI controller.
      mask init:
      | UpperLimit=Par_Limits(1);
      | LowerLimit=Par_Limits(2);
      | power_initmask();
      mask Help: This block is part of a subset of blocks in the Extras library that does not have documentation associated with it, other than the block mask description.
      mask Display: disp('PI');
  Discrete PI Controller3 : Subsystem  DialogController=POWERSYS.PowerSysDialog  mask(Discrete PI Controller){Kp=Kpv_buck, Ki=Kiv_buck, Par_Limits=[1 -1], Init=0, Ts=Tr_buck}
      mask prompts: Kp "Proportional gain (Kp):"; Ki "Integral gain (Ki):"; Par_Limits "Output limits: [ Upper   Lower ]"; Init "Output initial value:"; Ts "Sample time:"
      mask help: This block implements a discrete PI controller.
      mask init:
      | UpperLimit=Par_Limits(1);
      | LowerLimit=Par_Limits(2);
      | power_initmask();
      mask Help: This block is part of a subset of blocks in the Extras library that does not have documentation associated with it, other than the block mask description.
      mask Display: disp('PI');
  Discrete PI Controller4 : Subsystem  DialogController=POWERSYS.PowerSysDialog  mask(Discrete PI Controller){Kp=Kpi_buck, Ki=Kii_buck, Par_Limits=[1 -1], Init=0, Ts=Ts}
      mask prompts: Kp "Proportional gain (Kp):"; Ki "Integral gain (Ki):"; Par_Limits "Output limits: [ Upper   Lower ]"; Init "Output initial value:"; Ts "Sample time:"
      mask help: This block implements a discrete PI controller.
      mask init:
      | UpperLimit=Par_Limits(1);
      | LowerLimit=Par_Limits(2);
      | power_initmask();
      mask Help: This block is part of a subset of blocks in the Extras library that does not have documentation associated with it, other than the block mask description.
      mask Display: disp('PI');
  Divide : Product  Inputs=*/  SampleTime=Ts
  Divide1 : Product  Inputs=*/  SampleTime=Ts
  Divide2 : Product  Inputs=*/  SampleTime=Ts
  Multiply : Gain  Gain=-1
  Product : Product
  Product1 : Product  RndMeth=Zero
  Product3 : Product  RndMeth=Zero
  Product4 : Product
  Saturation : Saturate  UpperLimit=inf  LowerLimit=0.01  SampleTime=Ts
  Saturation Dynamic : simulink/Discontinuities/Saturation Dynamic  OutMin=[]  OutMax=[]  OutDataTypeStr=Inherit: Same as second input  OutDataType=fixdt(1, 16)  OutScaling=2^-10  DoSatur=off
  Saturation Dynamic1 : simulink/Discontinuities/Saturation Dynamic  OutMin=[]  OutMax=[]  OutDataTypeStr=Inherit: Same as second input  OutDataType=fixdt(1, 16)  OutScaling=2^-10  DoSatur=off
  Saturation1 : Saturate  UpperLimit=1  LowerLimit=0  SampleTime=Ts
  Saturation2 : Saturate  UpperLimit=inf  LowerLimit=0.01  SampleTime=Ts
  Saturation3 : Saturate  UpperLimit=1  LowerLimit=0  SampleTime=Ts
  Saturation4 : Saturate  UpperLimit=inf  LowerLimit=0.01  SampleTime=Ts
  Saturation6 : Saturate  UpperLimit=100  LowerLimit=0
  Saturation7 : Saturate  UpperLimit=100  LowerLimit=0
  Subsystem : Subsystem  Variant=on  VariantControlMode=label  VariantControl=Choice  LabelModeActiveChoice=Choice_1
  Sum{,1,8,10} (4 alike) : Sum  Inputs=|++
  Sum{2..4,7} (4 alike) : Sum  Inputs=|+-
  Sum5 : Sum  Inputs=|-+
  Sum6 : Sum  Inputs=|-+
  Sum9 : Sum  Inputs=+-
  R+ : PMIOPort  Side=Right
  L+ : PMIOPort  Port=2  Side=Left
  L- : PMIOPort  Port=3  Side=Left
  R- : PMIOPort  Port=4  Side=Right
  DutyCycle : Outport
  wires:
  I/O/1 -> [g]
  Discrete PI Controller3/1(Out) -> Sum4/1
  Sum3/1 -> Discrete PI Controller3/1(Error)
  Saturation Dynamic/1 -> Sum/1
  Sum/1 -> Discrete PI Controller4/1(Error)
  [IL] -> Sum/2
  [VBatt] -> Sum3/2
  Saturation/1 -> Divide/2
  Discrete PI Controller4/1(Out) -> Sum1/1
  Constant1/1 -> Saturation Dynamic/3
  Sum4/1 -> Saturation Dynamic/2
  [VBatt] -> Sum1/2
  Divide/1 -> Saturation1/1
  [Vdcbus] -> Saturation/1
  [Ibatt] -> Sum4/2
  Sum1/1 -> Divide/1
  Saturation1/1 -> Product/2
  converter/1 -> [converter]
  [converter] -> Product/1
  [Vdcbus] -> Saturation2/1
  [IL] -> Sum2/2
  Sum2/1 -> Discrete PI Controller2/1(Error)
  Constant/1 -> Sum6/2
  [VBatt] -> Sum5/2
  Sum5/1 -> Divide1/1
  [Vdcbus] -> Divide2/1
  Saturation Dynamic1/1 -> Sum2/1
  Constant2/1 -> Saturation Dynamic1/3
  [Vdcbus] -> Sum7/2
  Divide2/1 -> Product1/2
  Sum7/1 -> Discrete PI Controller1/1(Error)
  Product3/1 -> Saturation4/1
  [VBatt] -> Product3/1
  V*/1 -> Sum7/1, Sum3/1
  Sum8/1 -> Product1/1
  Product1/1 -> Saturation Dynamic1/2
  Sum6/1 -> Saturation3/1
  Discrete PI Controller1/1(Out) -> Sum8/1
  [Idcbus] -> Sum8/2
  Constant8/1 -> Product3/2
  Discrete PI Controller2/1(Out) -> Sum5/1
  Divide1/1 -> Sum6/1
  Saturation2/1 -> Divide1/2
  Saturation4/1 -> Divide2/2
  Saturation3/1 -> Product4/2
  Constant3/1 -> Sum9/1
  [converter] -> Sum9/2
  Sum9/1 -> Product4/1
  Product/1 -> Sum10/1
  Product4/1 -> Sum10/2
  Sum10/1 -> DutyCycle/1, [D]  "Duty Cycle BATT conv"
  Multiply/1 -> Saturation6/1
  Saturation6/1 -> Saturation Dynamic/1
  Saturation7/1 -> Saturation Dynamic1/1
  I*/1 -> Saturation7/1, Multiply/1
  [converter] -> Subsystem/3(converter)
  [g] -> Subsystem/1(g)
  [D] -> Subsystem/2(D)
  Subsystem/5(Vdcbus) -> [Vdcbus]
  Subsystem/4(Idcbus) -> [Idcbus]
  Subsystem/3(IL) -> [IL]
  Subsystem/2(Ibatt) -> [Ibatt]
  Subsystem/1(Vbatt) -> [VBatt]
  connections:
  L+/RConn1 -- Subsystem/LConn1
  L-/RConn1 -- Subsystem/LConn2
  R+/RConn1 -- Subsystem/RConn1
  R-/RConn1 -- Subsystem/RConn2
